simulink model "ARB_ACTIVE_PID."  (R2020a)
settings: Solver=FixedStepAuto  StartTime=0.0  StopTime=10  FixedStep=0.01  RelTol=1e-3
undefined symbols (not defined in the file or in its folder): A_ativo, B_ativo, D_ativo, sigbuilder_block
libraries: simulink x2
settings Model: Creator=Vitor  LastModifiedBy=Vitor
settings DebuggingCC: UnconnectedInputMsg=none  UnconnectedOutputMsg=none  UnconnectedLineMsg=none
settings ModelReferenceCC: EnableRefExpFcnMdlSchedulingChecks=off
settings RTWCC: Description=Generic Real-Time Target

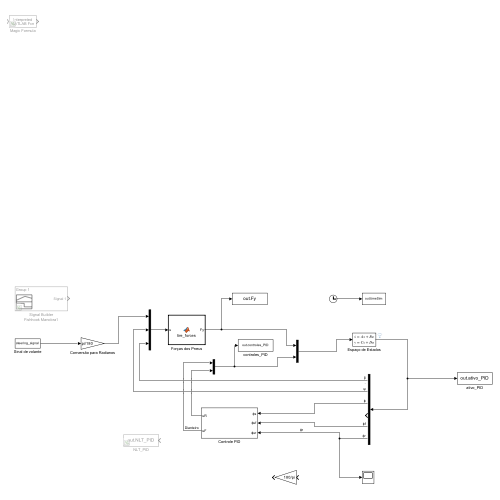
[thumbnail: Simulink's stored preview of the top-level diagram]
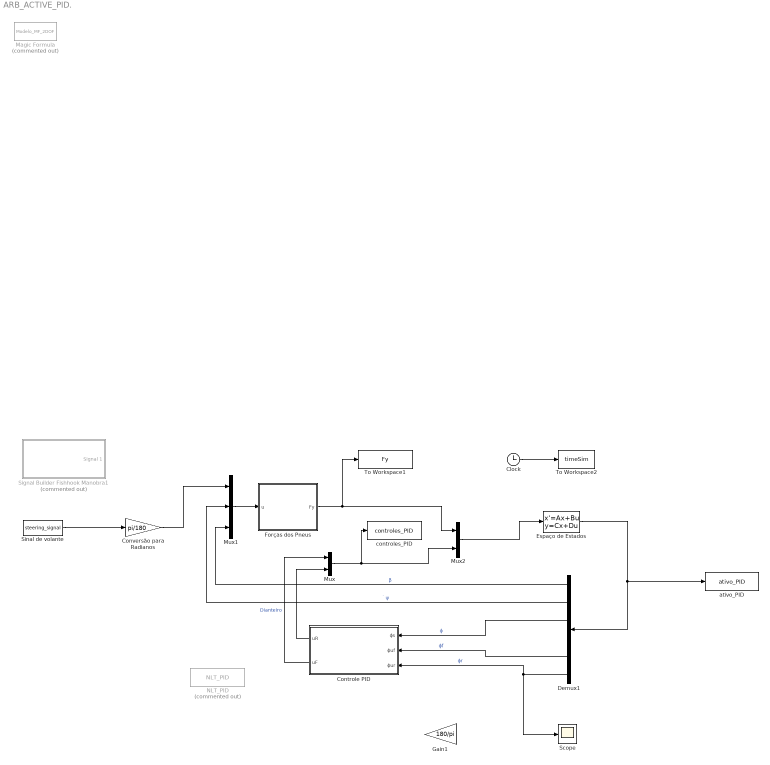
== system ARB_ACTIVE_PID. ==
  Clock : Clock
  Controle PID : Subsystem
  Conversão para Radianos : Gain  Gain=pi/180
  Demux1 : Demux  Outputs=6
  Espaço de Estados : StateSpace  A=A_ativo  B=B_ativo  C=eye(6)  D=D_ativo  InitialCondition=0
  Forças dos Pneus : MATLAB Function  TreatAsAtomicUnit=on
  Gain1 : Gain  Gain=180/pi
  Magic Formula : MATLABFcn  Commented=on  MATLABFcn=Modelo_MF_2DOF  OutputDimensions=2
  Mux : Mux  Inputs=2
  Mux1 : Mux  Inputs=3
  Mux2 : Mux  Inputs=2
  NLT_PID : ToWorkspace  Commented=on  VariableName=NLT_PID  SampleTime=-1
  Scope : Scope
  Signal Builder Fishhook Manobra1 : Subsystem  Tag=STV Subsys  Commented=on  LoadFcn=sigbuilder_block('load');  StartFcn=sigbuilder_block('start');  StopFcn=sigbuilder_block('stop');  ClipboardFcn=sigbuilder_block('clipboard');  mask(Sigbuilder block){tuvar=[0:10]}
      mask help: Simulink:masks:SigbuilderBlock_MD
      mask init:
      | if ~strcmp(get_param(bdroot(gcbh),'SimulationStatus'),'stopped') tuvar = sigbuilder_block('maskInit'); end
      settings: CopyFcn=sigbuilder_block('copy');  DeleteFcn=sigbuilder_block('delete');  ModelCloseFcn=sigbuilder_block('modelClose');  PreSaveFcn=sigbuilder_block('preSave');  PauseFcn=sigbuilder_block('pause');  ContinueFcn=sigbuilder_block('continue');  NameChangeFcn=sigbuilder_block('namechange');  OpenFcn=sigbuilder_block('open',[17.4 79.8 1141.2 438.6 ]);  CloseFcn=sigbuilder_block('close');
      mask Display: plot(0, 0, 100, 100,[2, 2, 32, 32, 2], [68, 8, 8, 68, 68],[32, 2], [38, 38], [32, 19, 2],[53, 60, 44], [32, 17, 17, 2],[16, 16, 31, 31]);txt = getActiveGroup(gcbh);text(2, 100, txt,'verticalAlignment', 'top');
  Sinal de volante : FromWorkspace  VariableName=steering_signal
  To Workspace1 : ToWorkspace  VariableName=Fy  SampleTime=-1
  To Workspace2 : ToWorkspace  VariableName=timeSim  SampleTime=-1
  ativo_PID : ToWorkspace  VariableName=ativo_PID  SampleTime=-1
  controles_PID : ToWorkspace  VariableName=controles_PID  SampleTime=-1
  wires:
  Sinal de volante/1 -> Conversão para Radianos/1
  Clock/1 -> To Workspace2/1
  Conversão para Radianos/1 -> Mux1/1
  Mux1/1 -> Forças dos Pneus/1(u)
  Demux1/2 -> Mux1/2  "˙ ψ"
  Demux1/1 -> Mux1/3  "β"
  Forças dos Pneus/1(Fy) -> To Workspace1/1, Mux2/1
  Espaço de Estados/1 -> Demux1/1, ativo_PID/1
  Demux1/5 -> Controle PID/2(ϕuf)  "ϕf"
  Demux1/6 -> Controle PID/3(ϕur), Scope/1  "ϕr"
  Controle PID/2(uF) -> Mux/1  "Dianteiro"
  Controle PID/1(uR) -> Mux/2
  Mux2/1 -> Espaço de Estados/1
  Mux/1 -> controles_PID/1, Mux2/2
  Demux1/3 -> Controle PID/1(ϕs)  "ϕ"

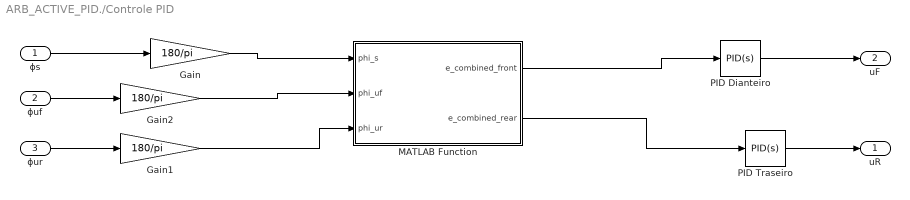
== system ARB_ACTIVE_PID./Controle PID ==
  ϕs : Inport
  ϕuf : Inport  Port=2
  ϕur : Inport  Port=3
  Gain : Gain  Gain=180/pi
  Gain1 : Gain  Gain=180/pi
  Gain2 : Gain  Gain=180/pi
  MATLAB Function : MATLAB Function  TreatAsAtomicUnit=on
  PID Dianteiro : simulink/Continuous/PID Controller  Controller=PID  Form=Parallel  TimeDomain=Continuous-time  UseExternalTs=off  SampleTime=-1  IntegratorMethod=Forward Euler  ControllerParametersSource=internal  P=1500  I=1200  D=50  N=100  UseFilter=on  TunerSelectOption=Transfer Function Based (PID Tuner App)  InitialConditionSource=internal  InitialConditionForIntegrator=0  InitialConditionForFilter=0  DifferentiatorICPrevScaledInput=0  ExternalReset=none  TrackingMode=off  Kt=1  LimitOutput=off  UpperSaturationLimit=inf  LowerSaturationLimit=-inf  LinearizeAsGain=on  AntiWindupMode=none  Kb=1  POutMin=[]  POutMax=[]  IOutMin=[]  IOutMax=[]  DOutMin=[]  DOutMax=[]  NOutMin=[]  NOutMax=[]  SumOutMin=[]  SumOutMax=[]  SaturationOutMin=[]  SaturationOutMax=[]  PParamMin=[]  PParamMax=[]  IParamMin=[]  IParamMax=[]  DParamMin=[]  DParamMax=[]  NParamMin=[]  NParamMax=[]  KbParamMin=[]  KbParamMax=[]  KtParamMin=[]  KtParamMax=[]  KbOutMin=[]  KbOutMax=[]  KtOutMin=[]  KtOutMax=[]  IntegratorOutMin=[]  IntegratorOutMax=[]  FilterOutMin=[]  FilterOutMax=[]  SumI1OutMin=[]  SumI1OutMax=[]  SumI2OutMin=[]  SumI2OutMax=[]  SumI3OutMin=[]  SumI3OutMax=[]  SumI4OutMin=[]  SumI4OutMax=[]  SumDOutMin=[]  SumDOutMax=[]  DifferentiatorOutMin=[]  DifferentiatorOutMax=[]  FilterDiffOutCoefMin=[]  FilterDiffOutCoefMax=[]  ReciprocalOutMin=[]  ReciprocalOutMax=[]  SumDenOutMin=[]  SumDenOutMax=[]  SumNumOutMin=[]  SumNumOutMax=[]  DivideOutMin=[]  DivideOutMax=[]  UdiffTsProdOutMin=[]  UdiffTsProdOutMax=[]  NTsProdOutMin=[]  NTsProdOutMax=[]  UintegralTsProdOutMin=[]  UintegralTsProdOutMax=[]  UngainTsProdOutMin=[]  UngainTsProdOutMax=[]  IntegratorContinuousStateAttributes=''  IntegratorStateMustResolveToSignalObject=off  IntegratorRTWStateStorageClass=Auto  FilterContinuousStateAttributes=''  FilterStateMustResolveToSignalObject=off  FilterRTWStateStorageClass=Auto  ParallelPVariant=InternalParameters  IdealPVariant=Disabled  IVariant=InternalParameters  DVariant=InternalParameters  IntegratorVariant=Continuous  SatVariant=Disabled  AWVariant=Passthrough  PCopyVariant=Disabled  TRVariant=Disabled  FdbkBlocksVariant=Forward  IdealPFdbkVariant=Disabled  SatFdbkVariant=Disabled  DerivativeFilterVariant=ContFilter  NVariant=InternalParameters  NCopyVariant=Disabled  FilterICVariant=InternalICsFilter  IntegratorICVariant=InternalICs  ExternalResetVariant=Disabled  TRSumVariant=Passthrough  SumFdbkVariant=Disabled  SumVariant=Sum_PID  TsampFilterVariant=InternalTs  TsampNgainVariant=Passthrough  TsampIntegralVariant=Disabled_SignalSpec
  PID Traseiro : simulink/Continuous/PID Controller  Controller=PID  Form=Parallel  TimeDomain=Continuous-time  UseExternalTs=off  SampleTime=-1  IntegratorMethod=Forward Euler  ControllerParametersSource=internal  P=1000  I=1500  D=75  N=100  UseFilter=on  TunerSelectOption=Transfer Function Based (PID Tuner App)  InitialConditionSource=internal  InitialConditionForIntegrator=0  InitialConditionForFilter=0  DifferentiatorICPrevScaledInput=0  ExternalReset=none  TrackingMode=off  Kt=1  LimitOutput=off  UpperSaturationLimit=inf  LowerSaturationLimit=-inf  LinearizeAsGain=on  AntiWindupMode=none  Kb=1  POutMin=[]  POutMax=[]  IOutMin=[]  IOutMax=[]  DOutMin=[]  DOutMax=[]  NOutMin=[]  NOutMax=[]  SumOutMin=[]  SumOutMax=[]  SaturationOutMin=[]  SaturationOutMax=[]  PParamMin=[]  PParamMax=[]  IParamMin=[]  IParamMax=[]  DParamMin=[]  DParamMax=[]  NParamMin=[]  NParamMax=[]  KbParamMin=[]  KbParamMax=[]  KtParamMin=[]  KtParamMax=[]  KbOutMin=[]  KbOutMax=[]  KtOutMin=[]  KtOutMax=[]  IntegratorOutMin=[]  IntegratorOutMax=[]  FilterOutMin=[]  FilterOutMax=[]  SumI1OutMin=[]  SumI1OutMax=[]  SumI2OutMin=[]  SumI2OutMax=[]  SumI3OutMin=[]  SumI3OutMax=[]  SumI4OutMin=[]  SumI4OutMax=[]  SumDOutMin=[]  SumDOutMax=[]  DifferentiatorOutMin=[]  DifferentiatorOutMax=[]  FilterDiffOutCoefMin=[]  FilterDiffOutCoefMax=[]  ReciprocalOutMin=[]  ReciprocalOutMax=[]  SumDenOutMin=[]  SumDenOutMax=[]  SumNumOutMin=[]  SumNumOutMax=[]  DivideOutMin=[]  DivideOutMax=[]  UdiffTsProdOutMin=[]  UdiffTsProdOutMax=[]  NTsProdOutMin=[]  NTsProdOutMax=[]  UintegralTsProdOutMin=[]  UintegralTsProdOutMax=[]  UngainTsProdOutMin=[]  UngainTsProdOutMax=[]  IntegratorContinuousStateAttributes=''  IntegratorStateMustResolveToSignalObject=off  IntegratorRTWStateStorageClass=Auto  FilterContinuousStateAttributes=''  FilterStateMustResolveToSignalObject=off  FilterRTWStateStorageClass=Auto  ParallelPVariant=InternalParameters  IdealPVariant=Disabled  IVariant=InternalParameters  DVariant=InternalParameters  IntegratorVariant=Continuous  SatVariant=Disabled  AWVariant=Passthrough  PCopyVariant=Disabled  TRVariant=Disabled  FdbkBlocksVariant=Forward  IdealPFdbkVariant=Disabled  SatFdbkVariant=Disabled  DerivativeFilterVariant=ContFilter  NVariant=InternalParameters  NCopyVariant=Disabled  FilterICVariant=InternalICsFilter  IntegratorICVariant=InternalICs  ExternalResetVariant=Disabled  TRSumVariant=Passthrough  SumFdbkVariant=Disabled  SumVariant=Sum_PID  TsampFilterVariant=InternalTs  TsampNgainVariant=Passthrough  TsampIntegralVariant=Disabled_SignalSpec
  uR : Outport
  uF : Outport  Port=2
  wires:
  ϕuf/1 -> Gain2/1
  ϕur/1 -> Gain1/1
  MATLAB Function/1(e_combined_front) -> PID Dianteiro/1
  MATLAB Function/2(e_combined_rear) -> PID Traseiro/1
  PID Dianteiro/1 -> uF/1
  PID Traseiro/1 -> uR/1
  Gain2/1 -> MATLAB Function/2(phi_uf)
  Gain1/1 -> MATLAB Function/3(phi_ur)
  ϕs/1 -> Gain/1
  Gain/1 -> MATLAB Function/1(phi_s)

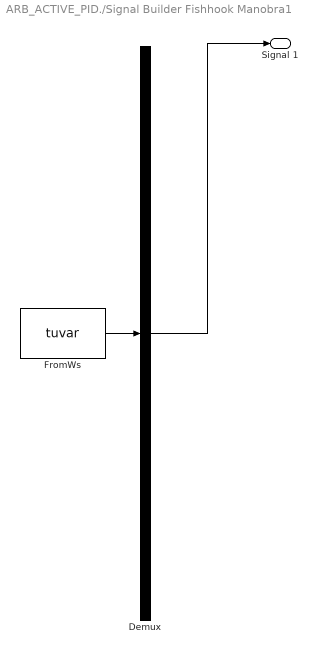
== system ARB_ACTIVE_PID./Signal Builder Fishhook Manobra1 ==
  Demux : Demux  Tag=STV Demux  Outputs=1
      settings: DisplayOption=none
  FromWs : FromWorkspace  Tag=STV FromWs  VariableName=tuvar
      SigBuilderData=|
      | common.afterFinalStr = 'Extrapolate'
      | common.sampleTime = 0
      | dataSet.timeRange = [0 10]
      | dataSet.name = 'Group 1'
      | sbobj.Groups.Name = 'Group 1'
      | sbobj.Groups.Signals.Name = 'Signal 1'
      | sbobj.Groups.Signals.XData = [0 1 1.25 1.5 2 5 9 10]
      | sbobj.Groups.Signals.YData = [0 0 10 10 -10 -10 0 0]
  Signal 1 : Outport  Tag=STV Outport
  wires:
  Demux/1 -> Signal 1/1
  FromWs/1 -> Demux/1

== matlab function ARB_ACTIVE_PID./Forças dos Pneus ==
  data: Fy output; u input
% Function: tire_forces.m
% Description: Calculate tire lateral forces using slip angles

function Fy  = tire_forces(u)
    % Descrição das Entradas
    beta = u(3);        % Ângulo de Deriva
    psi_dot = u(2);     % Taxa de Guinada
    delta_f = u(1);     % Ângulo de Esterçamento
    
    % Parâmetros do veículo (fixos na função para evitar problemas de escopo)
    lf = 1.95;           % Distância do CG ao eixo dianteiro (m)
    lr = 1.54;           % Distância do CG ao eixo traseiro (m)
    Cf = 582000;         % Rigidez lateral do pneu dianteiro (N/rad)
    Cr = 783000;         % Rigidez lateral do pneu traseiro (N/rad)
    mu = 1;              % Coeficiente de aderência ao solo
    v = 70 / 3.6;        % Velocidade longitudinal (m/s)
    
    % Calcular ângulos de deriva
    alpha_f = -beta + delta_f - ((lf * psi_dot) / v);
    alpha_r = -beta + ((lr * psi_dot) / v);
    
    % Calcular forças laterais nos pneus (saídas escalares)
    Fyf = mu * Cf * alpha_f;
    Fyr = mu * Cr * alpha_r;

    % Combinar as saídas como vetor coluna (2x1)
    Fy = [Fyf; Fyr];
end

== matlab function ARB_ACTIVE_PID./Controle PID/MATLAB Function ==
  data: phi_s input; phi_uf input; phi_ur input; e_combined_front output; e_combined_rear output
function [e_combined_front, e_combined_rear] = calcCombinedError(phi_s, phi_uf, phi_ur)
% Calcula o erro combinado para controle PID
% Entrada:
%   phi_s  - Ângulo de rolagem da massa suspensa (rad)
%   phi_uf - Ângulo de rolagem da massa não suspensa dianteira (rad)
%   phi_ur - Ângulo de rolagem da massa não suspensa traseira (rad)
%
% Saída:
%   e_combined_front - Erro para o PID do eixo dianteiro
%   e_combined_rear  - Erro para o PID do eixo traseiro

% Define pesos
w_susp    = 1;  % Peso da rolagem da massa suspensa (foco principal)
w_unsprung = 0.4; % Peso da rolagem das massas não suspensas (influência menor)

% Calcula erros individuais
e_phi_s = 0 - phi_s;   % Erro da massa suspensa
e_phi_uf = 0 - phi_uf; % Erro da não suspensa dianteira
e_phi_ur = 0 - phi_ur; % Erro da não suspensa traseira

% Combinação ponderada dos erros
e_combined_front = w_susp * e_phi_s + w_unsprung * e_phi_uf;
e_combined_rear  = w_susp * e_phi_s + w_unsprung * e_phi_ur;

end
